simulink model "Brake"  (R2022b)
settings: Solver=VariableStepAuto  StartTime=-2  StopTime=15  RelTol=1e-3
libraries: simulink x5, slpidlib x1
settings Model: Creator=david  LastModifiedBy=david
settings SolverCC: ZeroCrossAlgorithm=Adaptive
settings DebuggingCC: IgnoredZcDiagnostic=none  UnconnectedInputMsg=warning  UnconnectedOutputMsg=warning  UnconnectedLineMsg=warning
settings ModelReferenceCC: EnableRefExpFcnMdlSchedulingChecks=on
settings RTWCC: DLArmComputeVersion=19.05

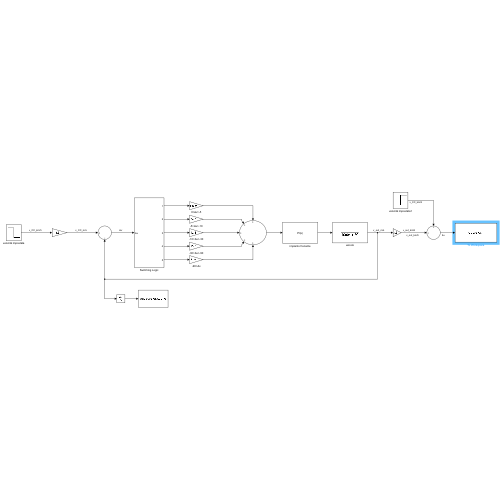
[thumbnail: Simulink's stored preview of the top-level diagram]
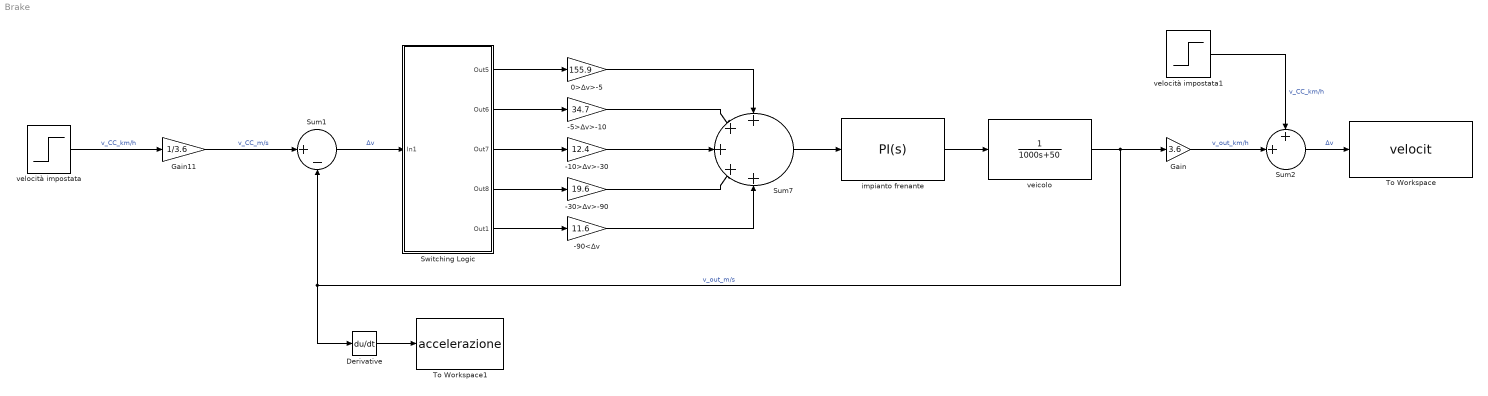
== system Brake ==
  -10>Δv>-30 : Gain  Gain=12.4
  -30>Δv>-90 : Gain  Gain=19.6
  -5>Δv>-10 : Gain  Gain=34.7
  -90<Δv : Gain  Gain=11.6
  0>Δv>-5 : Gain  Gain=155.9
  Derivative : Derivative
  Gain : Gain  Gain=3.6
  Gain11 : Gain  Gain=1/3.6
  Sum1 : Sum  Inputs=|+-
  Sum2 : Sum  Inputs=++|
  Sum7 : Sum  Inputs=+++++
  Switching Logic : Subsystem
  To Workspace : ToWorkspace  VariableName=velocit  SampleTime=-1
  To Workspace1 : ToWorkspace  VariableName=accelerazione  SampleTime=-1
  impianto frenante : slpidlib/PID Controller  Controller=PI  Form=Parallel  TimeDomain=Continuous-time  UseExternalTs=off  SampleTime=-1  IntegratorMethod=Forward Euler  FilterMethod=Forward Euler  ControllerParametersSource=internal  P=20  I=1  UseKiTs=off  D=0  N=100  UseFilter=on  TunerSelectOption=Transfer Function Based (PID Tuner App)  InitialConditionSource=internal  InitialConditionForIntegrator=0  InitialConditionForFilter=0  DifferentiatorICPrevScaledInput=0  ExternalReset=none  TrackingMode=off  Kt=1  LimitOutput=off  SatLimitsSource=internal  UpperSaturationLimit=inf  LowerSaturationLimit=-inf  LinearizeAsGain=on  AntiWindupMode=none  Kb=1  LimitIntegrator=off  UpperIntegratorSaturationLimit=inf  LowerIntegratorSaturationLimit=-inf  POutMin=[]  POutMax=[]  IOutMin=[]  IOutMax=[]  DOutMin=[]  DOutMax=[]  NOutMin=[]  NOutMax=[]  SumOutMin=[]  SumOutMax=[]  SaturationOutMin=[]  SaturationOutMax=[]  PParamMin=[]  PParamMax=[]  IParamMin=[]  IParamMax=[]  DParamMin=[]  DParamMax=[]  NParamMin=[]  NParamMax=[]  KbParamMin=[]  KbParamMax=[]  KtParamMin=[]  KtParamMax=[]  KbOutMin=[]  KbOutMax=[]  KtOutMin=[]  KtOutMax=[]  IntegratorOutMin=[]  IntegratorOutMax=[]  FilterOutMin=[]  FilterOutMax=[]  SumI1OutMin=[]  SumI1OutMax=[]  SumI2OutMin=[]  SumI2OutMax=[]  SumI3OutMin=[]  SumI3OutMax=[]  SumI4OutMin=[]  SumI4OutMax=[]  SumDOutMin=[]  SumDOutMax=[]  DifferentiatorOutMin=[]  DifferentiatorOutMax=[]  FilterDiffOutCoefMin=[]  FilterDiffOutCoefMax=[]  ReciprocalOutMin=[]  ReciprocalOutMax=[]  SumDenOutMin=[]  SumDenOutMax=[]  SumNumOutMin=[]  SumNumOutMax=[]  DivideOutMin=[]  DivideOutMax=[]  UdiffTsProdOutMin=[]  UdiffTsProdOutMax=[]  NTsProdOutMin=[]  NTsProdOutMax=[]  UintegralTsProdOutMin=[]  UintegralTsProdOutMax=[]  UngainTsProdOutMin=[]  UngainTsProdOutMax=[]  ClampingZeroOutDataTypeStr=Inherit: Inherit via back propagation  ClampingZeroOutMin=[]  ClampingZeroOutMax=[]  FilterDenConstantOutDataTypeStr=Inherit: Inherit via back propagation  FilterDenConstantOutMin=[]  FilterDenConstantOutMax=[]  PCopyOutDataTypeStr=Inherit: Inherit via back propagation  PCopyOutMin=[]  PCopyOutMax=[]  NCopyOutDataTypeStr=Inherit: Inherit via back propagation  NCopyOutMin=[]  NCopyOutMax=[]  IntegratorContinuousStateAttributes=''  IntegratorStateMustResolveToSignalObject=off  IntegratorRTWStateStorageClass=Auto  FilterContinuousStateAttributes=''  FilterStateMustResolveToSignalObject=off  FilterRTWStateStorageClass=Auto  ParallelPVariant=InternalParameters  IdealPVariant=Disabled  IVariant=InternalParameters  DVariant=Disabled  IntegratorVariant=Continuous  SatVariant=Disabled  AWVariant=Passthrough  PCopyVariant=Disabled  TRVariant=Disabled  FdbkBlocksVariant=Forward  IdealPFdbkVariant=Disabled  SatFdbkVariant=Disabled  DerivativeFilterVariant=Disabled  NVariant=Disabled  NCopyVariant=Disabled_SignalSpec  FilterICVariant=Disabled  IntegratorICVariant=InternalICs  ExternalResetVariant=Disabled  TRSumVariant=Passthrough  SumFdbkVariant=Disabled  SumVariant=Sum_PI  TsampFilterVariant=InternalTs  TsampNgainVariant=Passthrough  TsampIntegralVariant=Passthrough  ExternalSaturationOutDataTypeStr=Inherit: Same as second input
  veicolo : TransferFcn  Denominator=[1000 50]
  velocità impostata : Step  Time=0  After=-90  SampleTime=0.001
  velocità impostata1 : Step  Time=-2  After=90  SampleTime=0.0001
  wires:
  Derivative/1 -> To Workspace1/1
  impianto frenante/1 -> veicolo/1
  veicolo/1 -> Gain/1, Derivative/1, Sum1/2  "v_out_m/s"
  Gain11/1 -> Sum1/1  "v_CC_m/s"
  0>Δv>-5/1 -> Sum7/1
  -10>Δv>-30/1 -> Sum7/3
  -5>Δv>-10/1 -> Sum7/2
  -30>Δv>-90/1 -> Sum7/4
  velocità impostata/1 -> Gain11/1  "v_CC_km/h"
  Switching Logic/1(Out5) -> 0>Δv>-5/1
  Switching Logic/2(Out6) -> -5>Δv>-10/1
  Switching Logic/3(Out7) -> -10>Δv>-30/1
  Switching Logic/4(Out8) -> -30>Δv>-90/1
  Sum1/1 -> Switching Logic/1(In1)  "Δv"
  Sum7/1 -> impianto frenante/1
  Switching Logic/5(Out1) -> -90<Δv/1
  -90<Δv/1 -> Sum7/5
  Sum2/1 -> To Workspace/1  "Δv"
  velocità impostata1/1 -> Sum2/1  "v_CC_km/h"
  Gain/1 -> Sum2/2  "v_out_km/h"

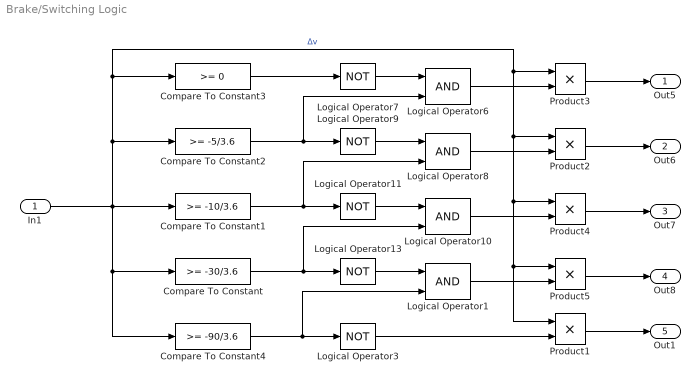
== system Brake/Switching Logic ==
  In1 : Inport
  Compare To Constant : simulink/Logic and Bit Operations/Compare To Constant  relop=>=  const=-30/3.6  OutDataTypeStr=boolean
  Compare To Constant1 : simulink/Logic and Bit Operations/Compare To Constant  relop=>=  const=-10/3.6  OutDataTypeStr=boolean
  Compare To Constant2 : simulink/Logic and Bit Operations/Compare To Constant  relop=>=  const=-5/3.6  OutDataTypeStr=boolean
  Compare To Constant3 : simulink/Logic and Bit Operations/Compare To Constant  relop=>=  const=0  OutDataTypeStr=boolean
  Compare To Constant4 : simulink/Logic and Bit Operations/Compare To Constant  relop=>=  const=-90/3.6  OutDataTypeStr=boolean
  Logical Operator{1,6,8,10} (4 alike) : Logic  AllPortsSameDT=off  OutDataTypeStr=boolean
  Logical Operator{3,7,9,11,13} (5 alike) : Logic  Operator=NOT  AllPortsSameDT=off  OutDataTypeStr=boolean
  Product{1..5} (5 alike) : Product
  Out5 : Outport
  Out6 : Outport  Port=2
  Out7 : Outport  Port=3
  Out8 : Outport  Port=4
  Out1 : Outport  Port=5
  wires:
  Logical Operator10/1 -> Product4/2
  Compare To Constant2/1 -> Logical Operator6/2, Logical Operator9/1
  Logical Operator11/1 -> Logical Operator10/1
  In1/1 -> Compare To Constant3/1, Product3/1, Product2/1, Product1/1, Product5/1, Product4/1, Compare To Constant2/1, Compare To Constant4/1, Compare To Constant/1, Compare To Constant1/1  "Δv"
  Logical Operator7/1 -> Logical Operator6/1
  Compare To Constant3/1 -> Logical Operator7/1
  Logical Operator13/1 -> Logical Operator1/1
  Logical Operator9/1 -> Logical Operator8/1
  Compare To Constant/1 -> Logical Operator10/2, Logical Operator13/1
  Compare To Constant1/1 -> Logical Operator8/2, Logical Operator11/1
  Logical Operator6/1 -> Product3/2
  Product5/1 -> Out8/1
  Product4/1 -> Out7/1
  Product2/1 -> Out6/1
  Product3/1 -> Out5/1
  Logical Operator8/1 -> Product2/2
  Compare To Constant4/1 -> Logical Operator1/2, Logical Operator3/1
  Logical Operator3/1 -> Product1/2
  Logical Operator1/1 -> Product5/2
  Product1/1 -> Out1/1
